simulink model "trajectory_generator_validation"  (R2015a)
settings: Solver=ode8  StartTime=0.0  StopTime=16  FixedStep=0.01  RelTol=1e-3
values from neighbouring files (symbols this model uses):
  J = 0.001118    [experiment1.mat]    (also in experiment2.mat; experiment3.mat; experiment4.mat; friction_ident.mat = 0.0001118)
  K = 0.053    [experiment1.mat]    (also in experiment2.mat; experiment3.mat; experiment4.mat; friction_ident.mat = 0.0053)
  max_voltage = 13.3    [experiment1.mat]    (also in experiment2.mat; experiment3.mat; experiment4.mat; friction_ident.mat)
  R = 2.71    [experiment1.mat]    (also in experiment2.mat; experiment3.mat; experiment4.mat; friction_ident.mat)
libraries: simulink x1
settings Model: Creator=Student  LastModifiedBy=Student

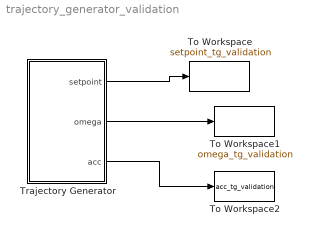
== system trajectory_generator_validation ==
  To Workspace : ToWorkspace  VariableName=setpoint_tg_validation  SampleTime=-1
  To Workspace1 : ToWorkspace  VariableName=omega_tg_validation  SampleTime=-1
  To Workspace2 : ToWorkspace  VariableName=acc_tg_validation  SampleTime=-1
  Trajectory Generator : Subsystem
  wires:
  Trajectory Generator/1(setpoint) -> To Workspace/1
  Trajectory Generator/2(omega) -> To Workspace1/1
  Trajectory Generator/3(acc) -> To Workspace2/1

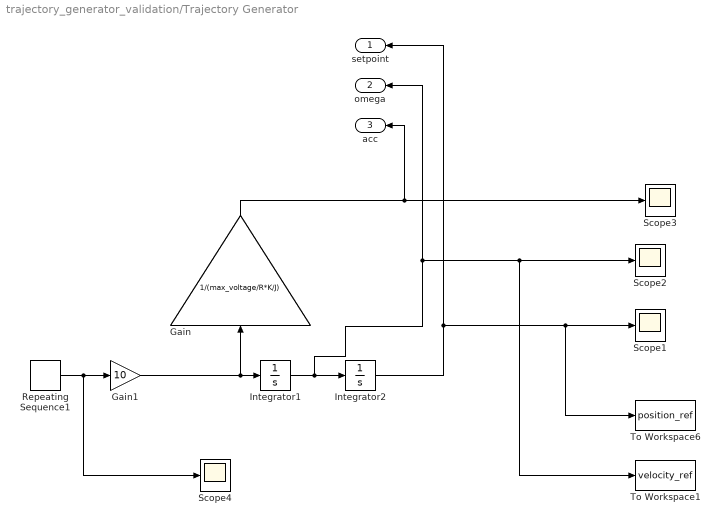
== system trajectory_generator_validation/Trajectory Generator ==
  Gain : Gain  Gain=1/(max_voltage/R*K/J)
  Gain1 : Gain  Gain=10
  Integrator1 : Integrator
  Integrator2 : Integrator
  Repeating Sequence1 : simulink/Sources/Repeating Sequence  rep_seq_t=repeat_time  rep_seq_y=repeat_val
  Scope{1..4} (4 alike) : Scope
      Scope1 settings: YMin=-0.008  YMax=-0.0045  SaveName=ScopeData9
      Scope2 settings: YMin=-110  YMax=90  SaveName=ScopeData8
      Scope3 settings: YMin=-0.22  YMax=0  SaveName=ScopeData10
      Scope4 settings: YMin=-0.22  YMax=0  SaveName=ScopeData11
  To Workspace1 : ToWorkspace  VariableName=velocity_ref  SampleTime=-1
  To Workspace6 : ToWorkspace  VariableName=position_ref  SampleTime=-1
  setpoint : Outport
  omega : Outport  Port=2
  acc : Outport  Port=3
  wires:
  Integrator2/1 -> To Workspace6/1, Scope1/1, setpoint/1
  Repeating Sequence1/1 -> Scope4/1, Gain1/1
  Integrator1/1 -> To Workspace1/1, Scope2/1, omega/1, Integrator2/1
  Gain/1 -> Scope3/1, acc/1
  Gain1/1 -> Gain/1, Integrator1/1
